simulink model "DSSDK_TrackerSingleObject"  (R2023a)
settings: Solver=FixedStepDiscrete  StartTime=0.0  StopTime=inf  RelTol=1e-3  EnableMultiTasking=on
settings Model: Creator=Ssubrama  LastModifiedBy=fedeoli
settings SolverCC: AlgebraicLoopSolver=TrustRegion
settings DataIOCC: LimitDataPoints=on  SaveFormat=Array  SignalLoggingSaveFormat=ModelDataLogs  ReturnWorkspaceOutputs=off
settings OptimizationCC: ExpressionDepthLimit=2147483647  InitFltsAndDblsToZero=on  LifeSpan=inf
settings DebuggingCC: UnderspecifiedInitializationDetection=Classic  MergeDetectMultiDrivingBlocksExec=none  SolverPrmCheckMsg=warning  FcnCallInpInsideContextMsg=warning  UnconnectedInputMsg=warning  UnconnectedOutputMsg=warning  UnconnectedLineMsg=warning  StateNameClashWarn=warning  SFUnexpectedBacktrackingDiag=warning  SFNoUnconditionalDefaultTransitionDiag=warning  SFExecutionAtInitializationDiag=none  ArithmeticOperatorsInVariantConditions=warning
settings HardwareCC: ProdBitPerPointer=32  ProdBitPerSizeT=32  ProdBitPerPtrDiffT=32  ProdLargestAtomicFloat=None  ProdIntDivRoundTo=Undefined  ProdEndianess=Unspecified  ProdWordSize=32  ProdHWDeviceType=32-bit Generic
settings ModelReferenceCC: PropagateSignalLabelsOutOfModel=off
settings SFSimCC: SimUseLocalCustomCode=off  CustomCodeUndefinedFunction=UseInterfaceOnly
settings RTWCC: RTWUseLocalCustomCode=off
settings CodeAppCC: StateflowObjectComments=on
settings GRTTargetCC: TargetFcnLib=ansi_tfl_tmw_new.mat  TargetLangStandard=C89/C90 (ANSI)  CombineOutputUpdateFcns=off  GRTInterface=on
settings ConfigComp: CovMetricSettings=dw  CovSaveCumulativeToWorkspaceVar=on  CovSaveSingleToWorkspaceVar=on  CovExternalEMLEnable=off  CovSFcnEnable=off

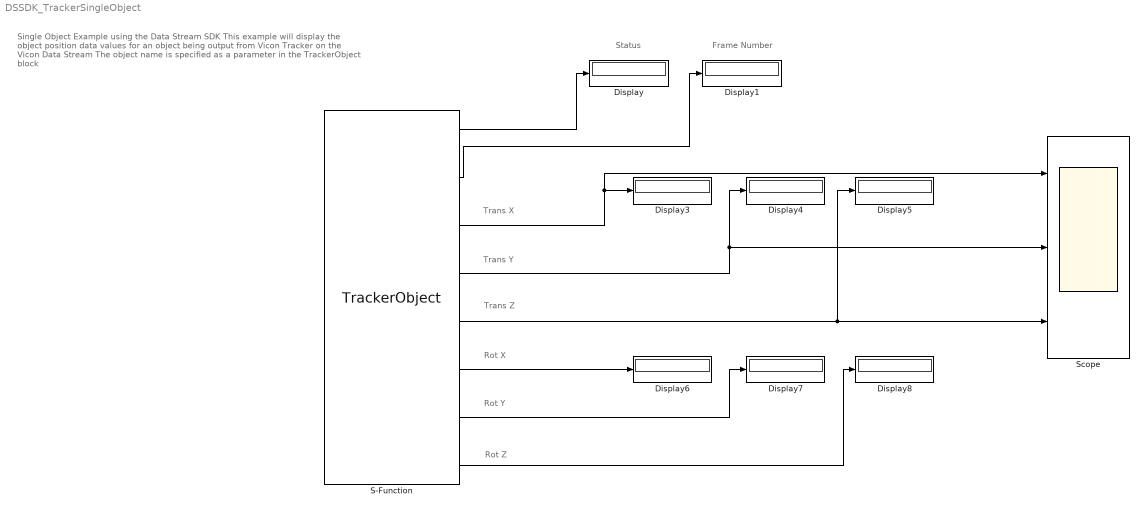
== system DSSDK_TrackerSingleObject ==
  note: Rot Z
  note: Rot Y
  note: Rot X
  note: Trans Z
  note: Trans Y
  note: Trans X
  note: Single Object Example
      | using the Data Stream SDK
      |
      | This example will display the object position data
      | values for an object being output from
      | Vicon Tracker on the Vicon Data Stream
      |
      | The object name is specified as a parameter
      | in the TrackerObject block
  note: Frame Number
  note: Status
  Display{,1,3..8} (8 alike) : Display
  S-Function : S-Function  FunctionName=TrackerObject  Parameters='CHEN'  SFunctionModules=TrackerObject  SFunctionDeploymentMode=off  EnableBusSupport=off
      settings: AttributesFormatString=Data Parser
  Scope : Scope  NumInputPorts=3
  wires:
  S-Function/1 -> Display/1
  S-Function/2 -> Display1/1
  S-Function/7 -> Display7/1
  S-Function/8 -> Display8/1
  S-Function/3 -> Scope/1, Display3/1
  S-Function/6 -> Display6/1
  S-Function/4 -> Display4/1, Scope/2
  S-Function/5 -> Display5/1, Scope/3
